simulink model "sm_car_testrig_bus_VehBusPower"  (R2020a)
settings: Solver=VariableStepAuto  StartTime=0.0  StopTime=10.0  RelTol=1e-3
undefined symbols (not defined in the file or in its folder): X, Y, Z
libraries: sm_lib x3, sm_car_lib x3, nesl_utility x2
Description:
  | Copyright 2020 The MathWorks, Inc.
settings Model: Creator=smiller  LastModifiedBy=smiller
settings DataIOCC: ReturnWorkspaceOutputs=off
settings DebuggingCC: ArithmeticOperatorsInVariantConditions=warning
settings SFSimCC: CustomCodeUndefinedFunction=UseInterfaceOnly
settings ExplorerConfigSet: SimMechanicsOpenEditorOnUpdate=off

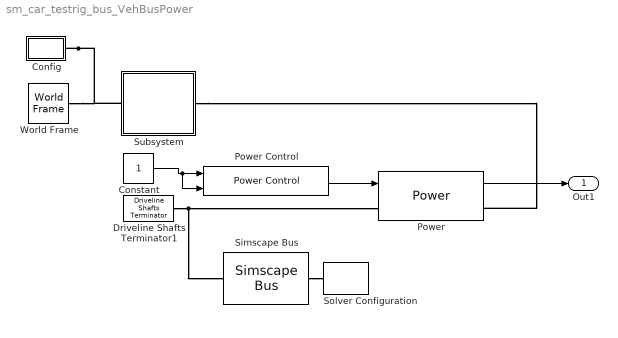
== system sm_car_testrig_bus_VehBusPower ==
  Config : Subsystem
  Constant : Constant
  Driveline Shafts Terminator1 : sm_car_lib/Driveline/Driveline Shafts Terminator  SystemSampleTime=-1  Latency=0  AutoFrameSizeCalculation=off
  Power : sm_car_lib/Power/Power  VariantControl=Variant1  LabelModeActiveChoice=Electric3Motor  Power=Vehicle.Powertrain.Power  VariantLabel=Vehicle.Powertrain.Power.class.Value  InitTriggerDropdown=1
      settings: AttributesFormatString=%<ActiveVariant>
  Power Control : sm_car_lib/Control/Power Control  trq_ratio_front=1
  Simscape Bus : SimscapeBus  HierarchyStrings=ShaftF
  Solver Configuration : nesl_utility/Solver Configuration  PhysicalDomain=network_engine_domain  SubClassName=solver  LeftPortType=input  RightPortType=generic  Tones=[]  Harmonics=[]  SimulateNoise=off  Profile=off  UseLocalSampling=off  EnableSwitchedLinearOptims=on  FrequencyDomain=off  UseCCode=off  RelTol=0.001  AbsTol=1e-06  MinStep=1e-09  ToWorkspace=off  RevertToSquareIcSolve=off  NumHomotopyIterations=100  PhasorMode=off  PhasorModeNumHarmonics=1  DoDC=off  ResidualTolerance=1e-09  UseLocalSolver=off  LocalSolverChoice=NE_BACKWARD_EULER_ADVANCER  LocalSolverSampleTime=0.001  DoFixedCost=off  MaxNonlinIter=3  MaxModeIter=2  LinearAlgebra=auto  EquationFormulation=NE_TIME_EF  DelaysMemoryBudget=1024  AutomaticFiltering=on  FilteringTimeConstant=0.001  PartitionStorageMethod=AS_NEEDED  PartitionMemoryBudget=1024  PartitionMethod=FAST
  Subsystem : Subsystem
  World Frame : sm_lib/Frames and Transforms/World Frame
  Out1 : Outport  OutDataTypeStr=Bus: VehiclePowerBusDef  VectorParamsAs1DForOutWhenUnconnected=off
      settings: AttributesFormatString=%<OutDataTypeStr>
  wires:
  Power Control/1 -> Power/1
  Power/1 -> Out1/1
  Constant/1 -> Power Control/2, Power Control/1
  connections:
  Config/RConn1 -- Subsystem/LConn1 -- World Frame/RConn1
  Driveline Shafts Terminator1/RConn1 -- Simscape Bus/RConn1 -- Power/LConn1
  Subsystem/RConn1 -- Power/RConn1
  Simscape Bus/LConn1 -- Solver Configuration/RConn1

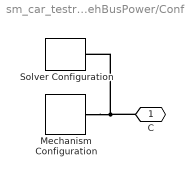
== system sm_car_testrig_bus_VehBusPower/Config ==
  Mechanism Configuration : sm_lib/Utilities/Mechanism Configuration  UniformGravity=Constant  GravityVector=[0 0 -9.80665]  GravityUnits=m/s^2  LinearizationDelta=0.001
  Solver Configuration : nesl_utility/Solver Configuration  PhysicalDomain=network_engine_domain  SubClassName=solver  LeftPortType=input  RightPortType=generic  Tones=[]  Harmonics=[]  SimulateNoise=off  Profile=off  UseLocalSampling=off  EnableSwitchedLinearOptims=on  FrequencyDomain=off  UseCCode=off  RelTol=0.001  AbsTol=1e-06  MinStep=1e-09  ToWorkspace=off  RevertToSquareIcSolve=off  NumHomotopyIterations=100  PhasorMode=off  PhasorModeNumHarmonics=1  DoDC=off  ResidualTolerance=1e-09  UseLocalSolver=off  LocalSolverChoice=NE_BACKWARD_EULER_ADVANCER  LocalSolverSampleTime=0.001  DoFixedCost=off  MaxNonlinIter=3  MaxModeIter=2  LinearAlgebra=Sparse  EquationFormulation=NE_TIME_EF  DelaysMemoryBudget=1024  AutomaticFiltering=on  FilteringTimeConstant=0.001  PartitionStorageMethod=AS_NEEDED  PartitionMemoryBudget=1024  PartitionMethod=FAST
  C : PMIOPort  Side=Right
  connections:
  Mechanism Configuration/RConn1 -- Solver Configuration/RConn1 -- C/RConn1

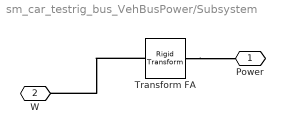
== system sm_car_testrig_bus_VehBusPower/Subsystem ==
  "Transform FA " : sm_lib/Frames and Transforms/Rigid Transform  TranslationMethod=Cartesian  TranslationStandardOffset=0  TranslationLengthUnit=m  TranslationStandardAxis=+Z  TranslationCartesianOffset=Vehicle.Chassis.Body.sAxleF.Value  TranslationROffset=0  TranslationROffsetUnits=m  TranslationZOffset=0  TranslationZOffsetUnits=m  TranslationThetaOffset=0  TranslationThetaOffsetUnits=deg  RotationMethod=None  RotationAngleUnits=deg  RotationStandardAxis=+Z  RotationAngle=0.0  RotationArbitraryAxis=[0 0 1]  FollAlignAxisA=+X  BaseAlignAxisA=+Y  FollAlignAxisB=+Y  BaseAlignAxisB=+Z  RotationSequenceAxes=FollowerAxes  RotationSequence=XYX  RotationSequenceAngles=[0 0 0]  RotationSequenceAnglesUnits=deg  RotationMatrix=[1 0 0; 0 1 0; 0 0 1]
  Power : PMIOPort  Side=Right
  W : PMIOPort  Port=2  Side=Left
  connections:
  "Transform FA "/LConn1 -- W/RConn1
  "Transform FA "/RConn1 -- Power/RConn1
